simulink library "modelLibrary"  (R2019b)
settings: Solver=VariableStepAuto  StartTime=0.0  StopTime=10.0  RelTol=1e-3
undefined symbols (not defined in the file or in its folder): Ks2, T7
settings Model: Creator=gdudgeon  LastModifiedBy=gdudgeon
settings DataIOCC: ReturnWorkspaceOutputs=off
settings DebuggingCC: PregeneratedLibrarySubsystemCodeDiagnostic=none  ArithmeticOperatorsInVariantConditions=warning
settings SFSimCC: SimUseLocalCustomCode=off  CustomCodeUndefinedFunction=UseInterfaceOnly
settings RTWCC: RTWUseLocalCustomCode=off

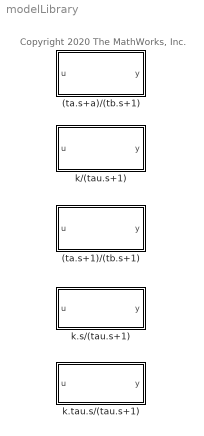
== system modelLibrary ==
  note: Copyright 2020 The MathWorks, Inc.
  (ta.s+1)/(tb.s+1) : Subsystem  mask{ta=1, tb=1}
      mask prompts: ta "numerator tau (ta)"; tb "denominator tau  (tb)"
  (ta.s+a)/(tb.s+1) : Subsystem  mask{ta=1, tb=1, a=1}
      mask prompts: ta "numerator tau (ta)"; tb "denominator tau  (tb)"
  k.s/(tau.s+1) : Subsystem  mask{k=1, tau=1}
  k.tau.s/(tau.s+1) : Subsystem  mask{k=1, tau=1}
  k/(tau.s+1) : Subsystem  mask{k=Ks2, tau=T7, vmax=Inf, vmin=-Inf}

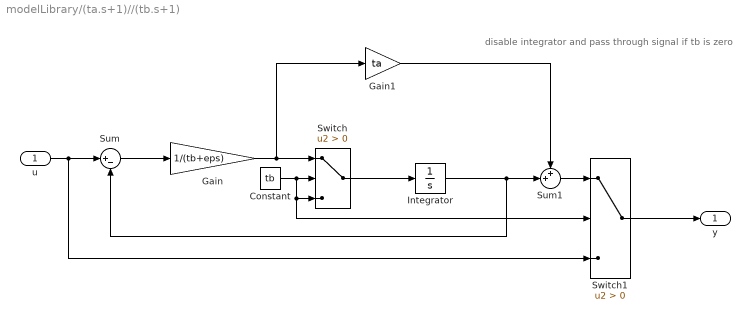
== system modelLibrary/(ta.s+1)//(tb.s+1) ==
  note: disable integrator and pass through signal if tb is zero
  u : Inport
  Constant : Constant  Value=tb
  Gain : Gain  Gain=1/(tb+eps)
  Gain1 : Gain  Gain=ta
  Integrator : Integrator
  Sum : Sum  Inputs=|+-
  Sum1 : Sum  Inputs=++|
  Switch : Switch  Criteria=u2 > Threshold
  Switch1 : Switch  Criteria=u2 > Threshold
  y : Outport  VectorParamsAs1DForOutWhenUnconnected=off
  wires:
  Sum/1 -> Gain/1
  Gain/1 -> Switch/1, Gain1/1
  Gain1/1 -> Sum1/1
  Integrator/1 -> Sum1/2, Sum/2
  u/1 -> Switch1/3, Sum/1
  Constant/1 -> Switch1/2, Switch/3, Switch/2
  Switch/1 -> Integrator/1
  Sum1/1 -> Switch1/1
  Switch1/1 -> y/1

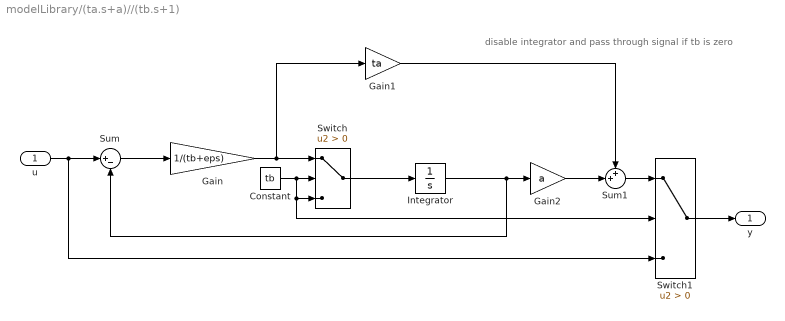
== system modelLibrary/(ta.s+a)//(tb.s+1) ==
  note: disable integrator and pass through signal if tb is zero
  u : Inport
  Constant : Constant  Value=tb
  Gain : Gain  Gain=1/(tb+eps)
  Gain1 : Gain  Gain=ta
  Gain2 : Gain  Gain=a
  Integrator : Integrator
  Sum : Sum  Inputs=|+-
  Sum1 : Sum  Inputs=++|
  Switch : Switch  Criteria=u2 > Threshold
  Switch1 : Switch  Criteria=u2 > Threshold
  y : Outport  VectorParamsAs1DForOutWhenUnconnected=off
  wires:
  Switch1/1 -> y/1
  Sum1/1 -> Switch1/1
  Switch/1 -> Integrator/1
  Constant/1 -> Switch/2, Switch/3, Switch1/2
  u/1 -> Sum/1, Switch1/3
  Integrator/1 -> Sum/2, Gain2/1
  Gain1/1 -> Sum1/1
  Gain/1 -> Gain1/1, Switch/1
  Sum/1 -> Gain/1
  Gain2/1 -> Sum1/2

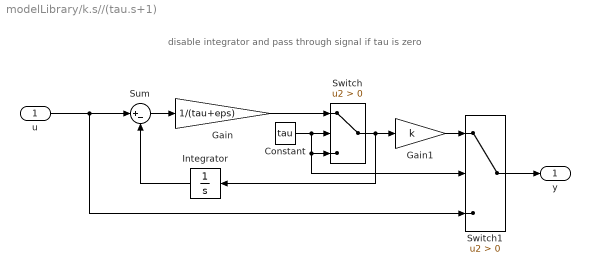
== system modelLibrary/k.s//(tau.s+1) ==
  note: disable integrator and pass through signal if tau is zero
  u : Inport
  Constant : Constant  Value=tau
  Gain : Gain  Gain=1/(tau+eps)
  Gain1 : Gain  Gain=k
  Integrator : Integrator
  Sum : Sum  Inputs=|+-
  Switch : Switch  Criteria=u2 > Threshold
  Switch1 : Switch  Criteria=u2 > Threshold
  y : Outport  VectorParamsAs1DForOutWhenUnconnected=off
  wires:
  Integrator/1 -> Sum/2
  u/1 -> Switch1/3, Sum/1
  Sum/1 -> Gain/1
  Constant/1 -> Switch1/2, Switch/3, Switch/2
  Gain/1 -> Switch/1
  Switch/1 -> Integrator/1, Gain1/1
  Switch1/1 -> y/1
  Gain1/1 -> Switch1/1

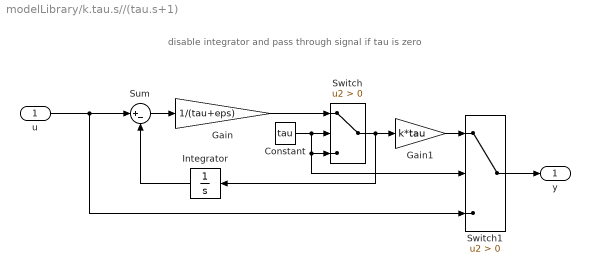
== system modelLibrary/k.tau.s//(tau.s+1) ==
  note: disable integrator and pass through signal if tau is zero
  u : Inport
  Constant : Constant  Value=tau
  Gain : Gain  Gain=1/(tau+eps)
  Gain1 : Gain  Gain=k*tau
  Integrator : Integrator
  Sum : Sum  Inputs=|+-
  Switch : Switch  Criteria=u2 > Threshold
  Switch1 : Switch  Criteria=u2 > Threshold
  y : Outport  VectorParamsAs1DForOutWhenUnconnected=off
  wires:
  Gain1/1 -> Switch1/1
  Switch1/1 -> y/1
  Switch/1 -> Gain1/1, Integrator/1
  Gain/1 -> Switch/1
  Constant/1 -> Switch/2, Switch/3, Switch1/2
  Sum/1 -> Gain/1
  u/1 -> Sum/1, Switch1/3
  Integrator/1 -> Sum/2

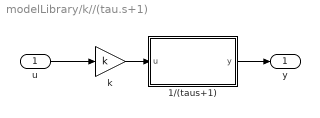
== system modelLibrary/k//(tau.s+1) ==
  u : Inport
  1/(taus+1) : Subsystem  mask{tau=tau, vmax=vmax, vmin=vmin}
      mask prompts: tau "Time Constant"
  k : Gain  Gain=k
  y : Outport  VectorParamsAs1DForOutWhenUnconnected=off
  wires:
  k/1 -> 1/(taus+1)/1(u)
  u/1 -> k/1
  1/(taus+1)/1(y) -> y/1

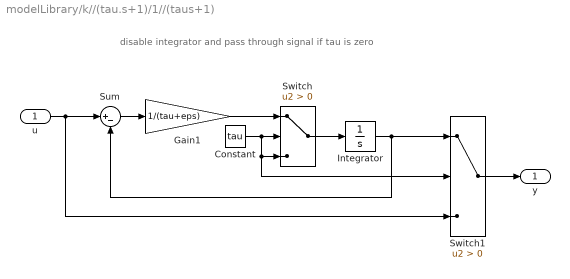
== system modelLibrary/k//(tau.s+1)/1//(taus+1) ==
  note: disable integrator and pass through signal if tau is zero
  u : Inport
  Constant : Constant  Value=tau
  Gain1 : Gain  Gain=1/(tau+eps)  SaturateOnIntegerOverflow=on  OutDataTypeStr=Inherit: Same as input  ParamDataTypeStr=Inherit: Same as input
  Integrator : Integrator  LimitOutput=on  UpperSaturationLimit=vmax  LowerSaturationLimit=vmin
  Sum : Sum  Inputs=|+-  SaturateOnIntegerOverflow=on  InputSameDT=on  OutDataTypeStr=Inherit: Same as first input
  Switch : Switch  Criteria=u2 > Threshold
  Switch1 : Switch  Criteria=u2 > Threshold
  y : Outport  VectorParamsAs1DForOutWhenUnconnected=off
  wires:
  u/1 -> Switch1/3, Sum/1
  Sum/1 -> Gain1/1
  Integrator/1 -> Sum/2, Switch1/1
  Constant/1 -> Switch/3, Switch1/2, Switch/2
  Gain1/1 -> Switch/1
  Switch/1 -> Integrator/1
  Switch1/1 -> y/1
